simulink model "sampleModel1707"  (R2023a)
settings: Solver=VariableStepAuto  StartTime=0.0  StopTime=10.0  RelTol=1e-3
libraries: hdlsllib x4, simulink x3
settings Model: Creator=user1  LastModifiedBy=user1

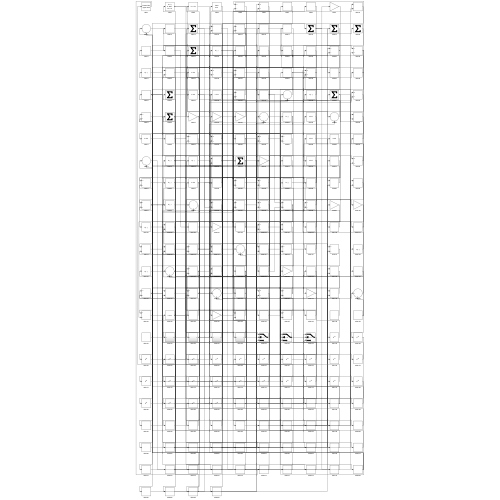
[thumbnail: Simulink's stored preview of the top-level diagram]
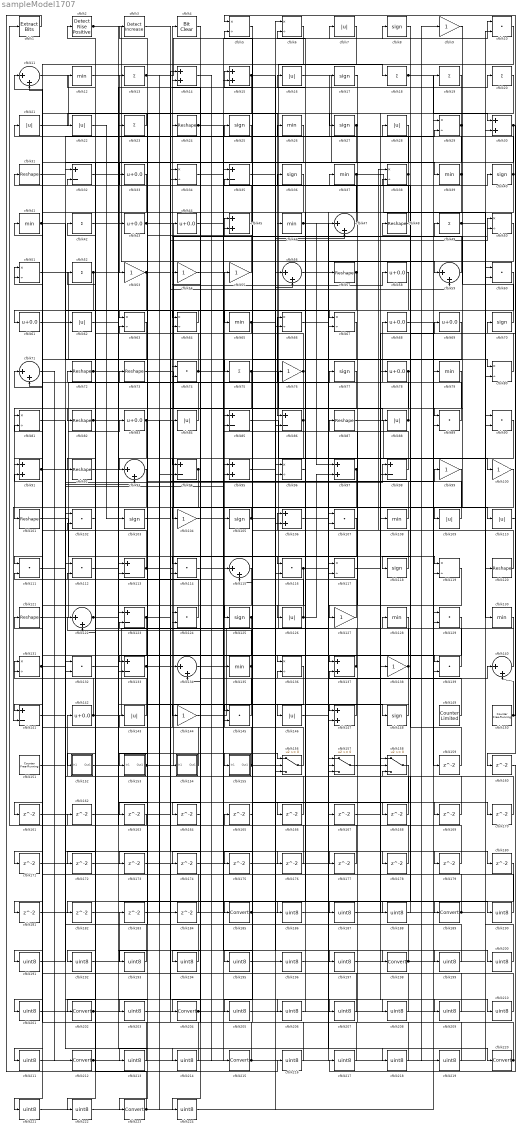
== system sampleModel1707 ==
  cfblk1 : simulink/Logic and Bit Operations/Extract Bits  bitsToExtract=Upper half  numBits=8  bitIdxRange=[0 7]  outScalingMode=Preserve fixed-point scaling
      settings: LibrarySourceBlock=|
      | hdlsllib/Logic and Bit
      | Operations/Extract Bits
  cfblk{10,60,74,89..90,102,107,111..112,114,116,124,129,132,139,145} (16 alike) : DotProduct  OutDataTypeStr=Inherit: Inherit via internal rule
  cfblk{9,53..55,76,99..100,104,127,138,144} (11 alike) : Gain
  cfblk{24,31,48,57,72..73,82,87,92,101,120..121} (12 alike) : Reshape
  cfblk{8,17,25,27,36,40,70,77,103,105,118,125,148} (13 alike) : Signum
  cfblk{14..15,30,45,91,95,97,106,137,147} (10 alike) : Sum
  cfblk{12,26,37,39,41,46,65,79,108,128,130,135} (12 alike) : MinMax
  cfblk{7,16,21..22,28,62,84,88,109..110,126,143,146} (13 alike) : Abs  SaturateOnIntegerOverflow=off
  cfblk{11,47,56,59,71,93,115,122,134,140} (10 alike) : Sum  Inputs=|++
  cfblk{32,35,85..86,94,98,113,123,133,141} (10 alike) : Sum  Inputs=+-
  cfblk{5..6,29,34,38,50..51,63..64,66..67,80..81,96,117,119,131,136} (18 alike) : Product  Inputs=*/  RndMeth=Zero  SaturateOnIntegerOverflow=on
  cfblk{13,18..20,23,42,49,52,75} (9 alike) : Sum  Inputs=+
  cfblk{33,43..44,58,61,68..69,78,83,142} (10 alike) : Bias  Bias=0.0  SaturateOnIntegerOverflow=off
  cfblk149 : hdlsllib/Sources/Counter Limited  uplimit=7  tsamp=-1
  cfblk150 : hdlsllib/Sources/Counter Free-Running  NumBits=16  tsamp=-1
  cfblk151 : hdlsllib/Sources/Counter Free-Running  NumBits=16  tsamp=-1
  cfblk152 : Subsystem
      settings: LibrarySourceBlock=|
      | hdlsllib/Ports &
      | Subsystems/Subsystem
  cfblk153 : Subsystem
      settings: LibrarySourceBlock=|
      | hdlsllib/Ports &
      | Subsystems/Subsystem
  cfblk154 : Subsystem
      settings: LibrarySourceBlock=|
      | hdlsllib/Ports &
      | Subsystems/Subsystem
  cfblk155 : Subsystem
      settings: LibrarySourceBlock=|
      | hdlsllib/Ports &
      | Subsystems/Subsystem
  cfblk156 : Switch  SaturateOnIntegerOverflow=off  InputSameDT=off
  cfblk157 : Switch  SaturateOnIntegerOverflow=off  InputSameDT=off
  cfblk158 : Switch  SaturateOnIntegerOverflow=off  InputSameDT=off
  cfblk{159..184} (26 alike) : Delay  SampleTime=1
  cfblk{185,189,198,202,204,212,215,220,223} (9 alike) : DataTypeConversion  SaturateOnIntegerOverflow=off  RndMeth=Floor
  cfblk{186..188,190..197,199..201,203,205..211,213..214,216..219,221..222,224} (31 alike) : DataTypeConversion  OutDataTypeStr=uint8  SaturateOnIntegerOverflow=off  RndMeth=Floor
  cfblk2 : hdlsllib/Logic and Bit Operations/Detect Rise Positive  vinit=0  OutDataTypeStr=boolean
  cfblk3 : simulink/Logic and Bit Operations/Detect Increase  vinit=0.0  OutDataTypeStr=boolean
      settings: LibrarySourceBlock=|
      | hdlsllib/Logic and Bit
      | Operations/Detect
      | Increase
  cfblk4 : simulink/Logic and Bit Operations/Bit Clear  iBit=0
      settings: LibrarySourceBlock=|
      | hdlsllib/Logic and Bit
      | Operations/Bit Clear
  wires:
  cfblk89/1 -> cfblk68/1
  cfblk125/1 -> cfblk163/1, cfblk191/1
  cfblk80/1 -> cfblk48/1
  cfblk18/1 -> cfblk9/1, cfblk30/1, cfblk219/1
  cfblk76/1 -> cfblk64/2, cfblk224/1
  cfblk13/1 -> cfblk7/1, cfblk184/1
  cfblk22/1 -> cfblk103/1
  cfblk142/1 -> cfblk18/1, cfblk131/1, cfblk156/2
  cfblk118/1 -> cfblk38/1
  cfblk155/1(Out1) -> cfblk55/1, cfblk23/1, cfblk187/1
  cfblk51/1 -> cfblk75/1
  cfblk21/1 -> cfblk86/1
  cfblk140/1 -> cfblk128/1
  cfblk96/1 -> cfblk142/1
  cfblk28/1 -> cfblk53/1
  cfblk109/1 -> cfblk36/1
  cfblk57/1 -> cfblk152/1(In1), cfblk175/1
  cfblk64/1 -> cfblk61/1
  cfblk133/1 -> cfblk58/1, cfblk156/1
  cfblk2/1 -> cfblk138/1, cfblk139/1
  cfblk150/1 -> cfblk5/1, cfblk140/2
  cfblk36/1 -> cfblk153/1(In1)
  cfblk158/1 -> cfblk185/1
  cfblk29/1 -> cfblk27/1, cfblk213/1
  cfblk121/1 -> cfblk83/1
  cfblk46/1 -> cfblk97/1, cfblk210/1
  cfblk151/1 -> cfblk98/1
  cfblk132/1 -> cfblk189/1
  cfblk88/1 -> cfblk72/1, cfblk11/2
  cfblk111/1 -> cfblk62/1
  cfblk45/1 -> cfblk13/1
  cfblk137/1 -> cfblk4/1, cfblk33/1
  cfblk74/1 -> cfblk137/1, cfblk52/1, cfblk10/1
  cfblk148/1 -> cfblk147/1
  cfblk105/1 -> cfblk104/1, cfblk170/1
  cfblk101/1 -> cfblk116/1
  cfblk34/1 -> cfblk105/1
  cfblk113/1 -> cfblk49/1, cfblk91/2, cfblk95/2
  cfblk32/1 -> cfblk96/1
  cfblk33/1 -> cfblk141/1
  cfblk70/1 -> cfblk45/1
  cfblk154/1(Out1) -> cfblk74/1
  cfblk23/1 -> cfblk22/1
  cfblk75/1 -> cfblk108/1, cfblk194/1
  cfblk116/1 -> cfblk50/1, cfblk181/1
  cfblk82/1 -> cfblk155/1(In1), cfblk172/1
  cfblk153/1(Out1) -> cfblk66/1, cfblk59/2
  cfblk6/1 -> cfblk204/1
  cfblk86/1 -> cfblk93/1, cfblk82/1
  cfblk98/1 -> cfblk45/2
  cfblk27/1 -> cfblk144/1, cfblk43/1
  cfblk71/1 -> cfblk212/1
  cfblk108/1 -> cfblk32/2
  cfblk47/1 -> cfblk37/1
  cfblk17/1 -> cfblk127/1
  cfblk5/1 -> cfblk125/1
  cfblk50/1 -> cfblk147/2
  cfblk126/1 -> cfblk85/1, cfblk97/2
  cfblk144/1 -> cfblk47/1
  cfblk54/1 -> cfblk198/1
  cfblk30/1 -> cfblk160/1, cfblk161/1
  cfblk43/1 -> cfblk135/1, cfblk94/2
  cfblk59/1 -> cfblk44/1
  cfblk138/1 -> cfblk111/2, cfblk186/1
  cfblk78/1 -> cfblk107/2, cfblk188/1
  cfblk85/1 -> cfblk100/1
  cfblk124/1 -> cfblk41/1
  cfblk87/1 -> cfblk120/1
  cfblk67/1 -> cfblk126/1
  cfblk122/1 -> cfblk77/1, cfblk146/1
  cfblk41/1 -> cfblk65/1, cfblk80/1, cfblk29/2
  cfblk55/1 -> cfblk3/1
  cfblk31/1 -> cfblk39/1
  cfblk112/1 -> cfblk24/1
  cfblk48/1 -> cfblk15/1
  cfblk94/1 -> cfblk122/2, cfblk182/1
  cfblk79/1 -> cfblk202/1
  cfblk14/1 -> cfblk215/1
  cfblk40/1 -> cfblk5/2, cfblk46/1
  cfblk127/1 -> cfblk106/1
  cfblk120/1 -> cfblk25/1
  cfblk11/1 -> cfblk154/1(In1)
  cfblk104/1 -> cfblk26/1
  cfblk24/1 -> cfblk119/1, cfblk67/2
  cfblk77/1 -> cfblk101/1
  cfblk58/1 -> cfblk114/1
  cfblk73/1 -> cfblk88/1
  cfblk91/1 -> cfblk15/2, cfblk93/2
  cfblk72/1 -> cfblk148/1, cfblk199/1
  cfblk83/1 -> cfblk113/2, cfblk106/2
  cfblk110/1 -> cfblk70/1
  cfblk37/1 -> cfblk130/1, cfblk59/1, cfblk94/1
  cfblk119/1 -> cfblk157/2
  cfblk49/1 -> cfblk60/2, cfblk109/1
  cfblk99/1 -> cfblk116/2
  cfblk20/1 -> cfblk98/2
  cfblk157/1 -> cfblk69/1
  cfblk139/1 -> cfblk31/1
  cfblk123/1 -> cfblk99/1, cfblk211/1
  cfblk147/1 -> cfblk21/1
  cfblk16/1 -> cfblk78/1
  cfblk145/1 -> cfblk73/1
  cfblk65/1 -> cfblk110/1, cfblk63/2
  cfblk8/1 -> cfblk118/1
  cfblk25/1 -> cfblk92/1
  cfblk134/1 -> cfblk40/1
  cfblk131/1 -> cfblk95/1, cfblk214/1
  cfblk90/1 -> cfblk133/1
  cfblk3/1 -> cfblk85/2
  cfblk130/1 -> cfblk123/2
  cfblk52/1 -> cfblk81/1, cfblk20/1
  cfblk35/1 -> cfblk47/2
  cfblk135/1 -> cfblk122/1, cfblk203/1
  cfblk146/1 -> cfblk140/1
  cfblk84/1 -> cfblk11/1
  cfblk10/1 -> cfblk64/1
  cfblk39/1 -> cfblk157/3, cfblk17/1
  cfblk60/1 -> cfblk63/1
  cfblk26/1 -> cfblk86/2
  cfblk97/1 -> cfblk141/2, cfblk156/3
  cfblk53/1 -> cfblk91/1, cfblk50/2
  cfblk149/1 -> cfblk124/1
  cfblk4/1 -> cfblk134/2
  cfblk143/1 -> cfblk51/1
  cfblk19/1 -> cfblk223/1
  cfblk61/1 -> cfblk28/1
  cfblk156/1 -> cfblk81/2
  cfblk15/1 -> cfblk34/2, cfblk111/1, cfblk178/1
  cfblk136/1 -> cfblk145/1
  cfblk9/1 -> cfblk89/1
  cfblk152/1(Out1) -> cfblk115/1
  cfblk114/1 -> cfblk8/1
  cfblk62/1 -> cfblk67/1
  cfblk56/1 -> cfblk220/1
  cfblk38/1 -> cfblk136/1, cfblk2/1
  cfblk68/1 -> cfblk159/1
  cfblk159/1 -> cfblk38/2
  cfblk161/1 -> cfblk133/2
  cfblk162/1 -> cfblk114/2
  cfblk163/1 -> cfblk1/1
  cfblk107/1 -> cfblk164/1
  cfblk164/1 -> cfblk74/2
  cfblk165/1 -> cfblk145/2
  cfblk92/1 -> cfblk166/1
  cfblk166/1 -> cfblk112/1
  cfblk66/1 -> cfblk168/1
  cfblk168/1 -> cfblk35/2
  cfblk44/1 -> cfblk169/1
  cfblk169/1 -> cfblk137/2
  cfblk170/1 -> cfblk123/1
  cfblk93/1 -> cfblk171/1
  cfblk171/1 -> cfblk157/1
  cfblk172/1 -> cfblk96/2
  cfblk100/1 -> cfblk173/1
  cfblk115/1 -> cfblk174/1
  cfblk103/1 -> cfblk176/1
  cfblk176/1 -> cfblk34/1
  cfblk141/1 -> cfblk177/1
  cfblk177/1 -> cfblk32/1
  cfblk178/1 -> cfblk136/2
  cfblk95/1 -> cfblk179/1
  cfblk179/1 -> cfblk113/1
  cfblk106/1 -> cfblk180/1
  cfblk181/1 -> cfblk119/2
  cfblk182/1 -> cfblk134/1
  cfblk183/1 -> cfblk90/1
  cfblk184/1 -> cfblk51/2
  cfblk185/1 -> cfblk115/2, cfblk57/1
  cfblk186/1 -> cfblk158/1
  cfblk187/1 -> cfblk158/2
  cfblk188/1 -> cfblk158/3
  cfblk189/1 -> cfblk124/2, cfblk107/1
  cfblk174/1 -> cfblk190/1
  cfblk190/1 -> cfblk132/1
  cfblk191/1 -> cfblk132/2
  cfblk102/1 -> cfblk192/1
  cfblk192/1 -> cfblk183/1
  cfblk128/1 -> cfblk193/1
  cfblk193/1 -> cfblk102/1
  cfblk194/1 -> cfblk102/2
  cfblk129/1 -> cfblk195/1
  cfblk195/1 -> cfblk90/2
  cfblk196/1 -> cfblk129/1
  cfblk175/1 -> cfblk197/1
  cfblk197/1 -> cfblk129/2
  cfblk198/1 -> cfblk10/2, cfblk143/1
  cfblk199/1 -> cfblk54/1
  cfblk167/1 -> cfblk200/1
  cfblk200/1 -> cfblk60/1
  cfblk63/1 -> cfblk201/1
  cfblk201/1 -> cfblk167/1
  cfblk202/1 -> cfblk80/2, cfblk66/2
  cfblk203/1 -> cfblk79/1
  cfblk204/1 -> cfblk89/2, cfblk76/1
  cfblk69/1 -> cfblk205/1
  cfblk205/1 -> cfblk6/1
  cfblk173/1 -> cfblk206/1
  cfblk206/1 -> cfblk6/2
  cfblk42/1 -> cfblk207/1
  cfblk207/1 -> cfblk16/1
  cfblk81/1 -> cfblk208/1
  cfblk208/1 -> cfblk42/1
  cfblk117/1 -> cfblk209/1
  cfblk209/1 -> cfblk121/1
  cfblk210/1 -> cfblk117/1
  cfblk211/1 -> cfblk117/2
  cfblk212/1 -> cfblk30/2, cfblk35/1
  cfblk213/1 -> cfblk71/1
  cfblk214/1 -> cfblk71/2
  cfblk215/1 -> cfblk196/1, cfblk131/2, cfblk139/2
  cfblk1/1 -> cfblk216/1
  cfblk216/1 -> cfblk14/1
  cfblk160/1 -> cfblk217/1
  cfblk217/1 -> cfblk14/2
  cfblk12/1 -> cfblk218/1
  cfblk218/1 -> cfblk112/2
  cfblk219/1 -> cfblk12/1
  cfblk220/1 -> cfblk165/1, cfblk29/1, cfblk87/1
  cfblk7/1 -> cfblk221/1
  cfblk221/1 -> cfblk56/1
  cfblk180/1 -> cfblk222/1
  cfblk222/1 -> cfblk56/2
  cfblk223/1 -> cfblk162/1, cfblk84/1
  cfblk224/1 -> cfblk19/1

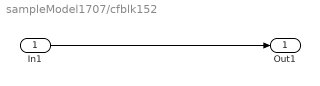
== system sampleModel1707/cfblk152 ==
  In1 : Inport
  Out1 : Outport
  wires:
  In1/1 -> Out1/1

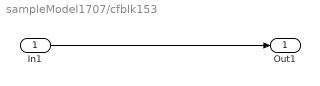
== system sampleModel1707/cfblk153 ==
  In1 : Inport
  Out1 : Outport
  wires:
  In1/1 -> Out1/1

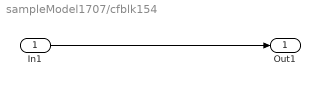
== system sampleModel1707/cfblk154 ==
  In1 : Inport
  Out1 : Outport
  wires:
  In1/1 -> Out1/1

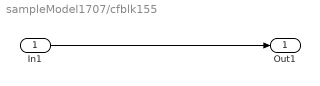
== system sampleModel1707/cfblk155 ==
  In1 : Inport
  Out1 : Outport
  wires:
  In1/1 -> Out1/1
